simulink model "M10B39_es_V3"  (R2025a)
settings: Solver=ode23tb  StartTime=0.0  StopTime=100  FixedStep=0.001  MaxStep=0.01  RelTol=1e-3  EnableMultiTasking=on
InitFcn:
  | initAll_V3
values from neighbouring files (symbols this model uses):
  acom = 100    [initAll_V1.m]    (also in initAll_V2.m; initAll_V3.m; parameterinit.mat)
  AVm0 = [4.26082678503 4.656135219]    [parameterinit.mat]
  bcom = 50    [initAll_V1.m]    (also in initAll_V2.m; initAll_V3.m; parameterinit.mat)
  commun = 0*commun    [initAll_V1.m]    (also in initAll_V2.m; initAll_V3.m; parameterinit.mat = [0  0  0; 0  0  0; 0  0  0; 0  0  0])
  DataDelay = 0.0*DataDelay    [initAll_V1.m]    (also in initAll_V2.m; initAll_V3.m; parameterinit.mat = [0  0  0; 0  0  0; 0  0  0; 0  0  0])
  ESinit =     [parameterinit.mat]
  fB = 50    [initAll.m]    (also in initAll_V1.m; initAll_V2.m; initAll_V3.m; parameterinit.mat)
  Geninit = Generator_init(opdata,SynMach_in_gidx)    [initAll.m]    (also in initAll_V1.m; initAll_V2.m; initAll_V3.m = Generator_init(opdata_all,SynMach_in_gidx1); parameterinit.mat = )
  lam = 100    [initAll_V1.m]    (also in initAll_V2.m; initAll_V3.m; parameterinit.mat)
  SgridB = 100    [initAll.m]    (also in initAll_V1.m; initAll_V2.m; initAll_V3.m; parameterinit.mat)
  wB = 2*pi*fB    (= 314.159265359)    [initAll.m]    (also in initAll_V1.m; initAll_V2.m; initAll_V3.m; parameterinit.mat)
  Windinit =     [parameterinit.mat]
  YY_load = [3.65450097002 -2.05705688056 0 0 0 0 0 0 0 0 0 0 ... (1521 elements, 39x39)]    [parameterinit.mat]    (also in powerflowcaculate.m = full(YY))
undefined symbols (not defined in the file or in its folder): c1, c2, c3, c4, c5, c6, cp_nom, lambda_nom, P_wind_base, Pelec_base, Pnom
libraries: spsBistableLib x12, simulink_extras x3, slpidlib x2, simulink x1
(part 4 of 7)

== system M10B39_es_V3/Genrators/Generator1/Governor ==
  w : Inport
  Trip : Inport  Port=2
  CT : Constant  Value=0
  Constant : Constant  Value=0
  Gain : Gain  Gain=a_G  SaturateOnIntegerOverflow=on  OutDataTypeStr=Inherit: Same as input  ParamDataTypeStr=Inherit: Same as input
  Saturation : Saturate  UpperLimit=dPmax  LowerLimit=dPmin
  Sum1 : Sum  Inputs=|++  SaturateOnIntegerOverflow=on
  Sum3 : Sum  Inputs=|+-  SaturateOnIntegerOverflow=on
  Switch : Switch  Threshold=0.5  InputSameDT=off
  Switch1 : Switch  Criteria=u2 ~= 0  Threshold=0.5  InputSameDT=off
  Transfer Fcn1 : TransferFcn  Numerator=[b_G]  Denominator=[Tg_G 1]
  w0 : Gain  Gain=wB  SaturateOnIntegerOverflow=on  OutDataTypeStr=Inherit: Same as input  ParamDataTypeStr=Inherit: Same as input
  w1 : Constant  Value=S_Gov
  wref : Constant
  dPm : Outport
  wires:
  Gain/1 -> Sum1/1
  w1/1 -> Switch/2
  CT/1 -> Switch/3
  Sum3/1 -> w0/1
  Sum1/1 -> Saturation/1
  Saturation/1 -> Switch/1
  wref/1 -> Sum3/1
  w0/1 -> Gain/1, Transfer Fcn1/1
  Transfer Fcn1/1 -> Sum1/2
  w/1 -> Sum3/2
  Constant/1 -> Switch1/1
  Switch/1 -> Switch1/3
  Trip/1 -> Switch1/2
  Switch1/1 -> dPm/1

== system M10B39_es_V3/Genrators/Generator1/Machine Equations  ==
  note: Iqg
  note: Idg
  note: 接口
  delta : Inport
  Vgxy : Inport  Port=2
  Ef : Inport  Port=3
  Trip : Inport  Port=4
  Demux : Demux  Outputs=2
  Demux1 : Demux  Outputs=2
  Fcn1 : Fcn  Expr=u(1)*u(3)+u(2)*u(4)
  Fcn2 : Fcn  Expr=(u(3)-u(2))/Xd1
  Fcn3 : Fcn  Expr=(u(1)-u(4))/Xq1
  Fcn4 : Fcn  Expr=u(2)*u(3)-u(1)*u(4)
  Fcn6 : Fcn  Expr=sqrt(u(1)^2+u(2)^2)
  Interface : Subsystem
  Mux1 : Mux  Inputs=2
  Mux2 : Mux  Inputs=2
  Mux3 : Mux  Inputs=2
  Qe : Scope
      settings: TimeSpan=10  ActiveDisplayYMinimum=0.15  ActiveDisplayYMaximum=0.65
  Scope{,1..3} (4 alike) : Scope
      Scope settings: ActiveDisplayYMinimum=6.90941  ActiveDisplayYMaximum=6.93032
      Scope1 settings: ActiveDisplayYMinimum=0.73198  ActiveDisplayYMaximum=0.74189  DataLoggingVariableName=ScopeData2
      Scope2 settings: ActiveDisplayYMinimum=0.70724  ActiveDisplayYMaximum=0.71179  DataLoggingVariableName=ScopeData3
      Scope3 settings: ActiveDisplayYMinimum=3.59596  ActiveDisplayYMaximum=3.95434  DataLoggingVariableName=ScopeData4
  Transient Equations : Subsystem
  Pe : Outport
  Igxy1 : Outport  Port=2
  GBxy : Outport  Port=3
  Vg : Outport  Port=4
  wires:
  Trip/1 -> Transient Equations/3(Trip)
  Demux1/2 -> Scope3/1
  Demux/2 -> Scope2/1
  Demux1/1 -> Scope/1
  Demux/1 -> Scope1/1
  Transient Equations/1(Eqd') -> Interface/3(Eqd''), Mux1/2
  Interface/3(GBxy) -> GBxy/1
  Interface/2(Igxy1) -> Igxy1/1
  Vgxy/1 -> Interface/2(Vgxy)
  delta/1 -> Interface/1(delta)
  Fcn4/1 -> Qe/1
  Fcn6/1 -> Vg/1
  Fcn1/1 -> Pe/1
  Ef/1 -> Transient Equations/2(Ef)
  Mux2/1 -> Fcn4/1, Fcn1/1
  Mux1/1 -> Fcn3/1, Fcn2/1
  Interface/1(Vdqg) -> Mux1/1, Fcn6/1, Mux2/1, Demux/1
  Mux3/1 -> Mux2/2, Demux1/1, Transient Equations/1(Idqg)
  Fcn2/1 -> Mux3/1
  Fcn3/1 -> Mux3/2

== system M10B39_es_V3/Genrators/Generator1/Mechanical DE ==
  Pe : Inport
  dPm : Inport  Port=2
  Trip : Inport  Port=3
  Constant1 : Constant  Value=0
  Constant2 : Constant  Value=0
  Gain : Gain  Gain=wB  SaturateOnIntegerOverflow=on  OutDataTypeStr=Inherit: Same as input  ParamDataTypeStr=Inherit: Same as input
  Gain1 : Gain  Gain=1/H  SaturateOnIntegerOverflow=on  OutDataTypeStr=Inherit: Same as input  ParamDataTypeStr=Inherit: Same as input
  Gain2 : Gain  Gain=D  SaturateOnIntegerOverflow=on  OutDataTypeStr=Inherit: Same as input  ParamDataTypeStr=Inherit: Same as input
  Gain5 : Gain  Gain=180/pi  SaturateOnIntegerOverflow=on  OutDataTypeStr=Inherit: Same as input  ParamDataTypeStr=Inherit: Same as input
  Int1 : Integrator  InitialCondition=delta0
  Int2 : Integrator  InitialCondition=w0
  Pm : Constant  Value=Pm0
  Scope2 : Scope
      settings: TimeSpan=10  ActiveDisplayYMinimum=-0.4  ActiveDisplayYMaximum=1.4  DataLoggingVariableName=ScopeData5
  Scope4 : Scope
      settings: TimeSpan=10  ActiveDisplayYMinimum=0.99397  ActiveDisplayYMaximum=1.02044  DataLoggingVariableName=ScopeData6
  Scope8 : Scope
      settings: TimeSpan=10  ActiveDisplayYMinimum=-0.4  ActiveDisplayYMaximum=1.4  DataLoggingVariableName=ScopeData11
  Sum2 : Sum  Inputs=-+-+  SaturateOnIntegerOverflow=on
  Sum3 : Sum  Inputs=|+-  SaturateOnIntegerOverflow=on
  Switch{1..4} (4 alike) : Switch  Criteria=u2 ~= 0  Threshold=0.5  InputSameDT=off
  w0 : Constant
  delta : Outport
  w : Outport  Port=2
  wires:
  [Trip] -> Switch3/2, Switch2/2
  Constant1/1 -> Switch3/1, Switch2/1
  Switch3/1 -> Scope4/1, Sum3/1, w/1
  Int2/1 -> Switch3/3
  Switch2/1 -> Int2/1
  Gain1/1 -> Switch2/3
  Trip/1 -> [Trip]
  [Trip] -> Switch1/2, Switch4/2
  Constant2/1 -> Switch4/1, Switch1/1
  Switch4/1 -> delta/1, Scope2/1, Gain5/1
  Int1/1 -> Switch4/3
  Switch1/1 -> Int1/1
  Gain/1 -> Switch1/3
  Gain5/1 -> Scope8/1
  w0/1 -> Sum3/2
  Sum3/1 -> Gain2/1, Gain/1
  Pm/1 -> Sum2/2
  Gain2/1 -> Sum2/1
  Sum2/1 -> Gain1/1
  Pe/1 -> Sum2/3
  dPm/1 -> Sum2/4

== system M10B39_es_V3/Genrators/Generator1/Output ==
  Igxy1in : Inport
  GBxyin : Inport  Port=2
  deltain : Inport  Port=3
  Pein : Inport  Port=4
  fin : Inport  Port=5
  Vg : Inport  Port=6
  Bus Creator : BusCreator  Inputs=6
  m : Outport
  Igxy1 : Outport  Port=2
  GBxy : Outport  Port=3
  wires:
  Vg/1 -> Bus Creator/6  "Vg"
  fin/1 -> Bus Creator/5  "f"
  Pein/1 -> Bus Creator/4  "Pe"
  deltain/1 -> Bus Creator/3  "delta"
  GBxyin/1 -> Bus Creator/2, GBxy/1  "GBxy"
  Igxy1in/1 -> Bus Creator/1, Igxy1/1  "Igxy1"
  Bus Creator/1 -> m/1

== system M10B39_es_V3/Genrators/Generator1/PSS1 ==
  w : Inport
  Trip : Inport  Port=2
  CT : Constant  Value=0
  Constant : Constant  Value=0
  Gain : Gain  Gain=Kpss  SaturateOnIntegerOverflow=on  OutDataTypeStr=Inherit: Same as input  ParamDataTypeStr=Inherit: Same as input
  Saturation : Saturate  UpperLimit=Upmax  LowerLimit=Upmin
  Sum3 : Sum  Inputs=|+-  SaturateOnIntegerOverflow=on
  Switch : Switch  Threshold=0.5  InputSameDT=off
  Switch1 : Switch  Threshold=0.5  InputSameDT=off
  Transfer Fcn : TransferFcn  Numerator=[Tw_P 0]  Denominator=[Tw_P 1]
  Transfer Fcn1 : TransferFcn  Numerator=[T1_P 1]  Denominator=[T2_P 1]
  Transfer Fcn2 : TransferFcn  Numerator=[T3_P 1]  Denominator=[T4_P 1]
  w0 : Constant
  w1 : Constant  Value=S_PSS
  Upss : Outport
  wires:
  Constant/1 -> Switch1/1
  Trip/1 -> Switch1/2
  Switch1/1 -> Upss/1
  Switch/1 -> Switch1/3
  Transfer Fcn/1 -> Transfer Fcn1/1
  Gain/1 -> Transfer Fcn/1
  w1/1 -> Switch/2
  CT/1 -> Switch/3
  Saturation/1 -> Switch/1
  Sum3/1 -> Gain/1
  Transfer Fcn2/1 -> Saturation/1
  Transfer Fcn1/1 -> Transfer Fcn2/1
  w/1 -> Sum3/1
  w0/1 -> Sum3/2

== system M10B39_es_V3/Genrators/Generator10/Excitation System ST1A1 ==
  note: Ef
  Upss : Inport
  Trip : Inport  Port=2
  Vg : Inport  Port=3
  Constant1 : Constant  Value=0
  Ef1 : Integrator  InitialCondition=Ef10
  K : Gain  Gain=1/Tb  SaturateOnIntegerOverflow=on  OutDataTypeStr=Inherit: Same as input  ParamDataTypeStr=Inherit: Same as input
  KA : Gain  Gain=Ka  SaturateOnIntegerOverflow=on  OutDataTypeStr=Inherit: Same as input  ParamDataTypeStr=Inherit: Same as input
  KA1 : Gain  Gain=Tc/Tb  SaturateOnIntegerOverflow=on  OutDataTypeStr=Inherit: Same as input  ParamDataTypeStr=Inherit: Same as input
  KA2 : Gain  Gain=(1/Tb)*(1-Tc/Tb)  SaturateOnIntegerOverflow=on  OutDataTypeStr=Inherit: Same as input  ParamDataTypeStr=Inherit: Same as input
  Saturation : Saturate  UpperLimit=Efmax  LowerLimit=Efmin
  Sum : Sum  Inputs=|++  SaturateOnIntegerOverflow=on
  Sum1 : Sum  Inputs=|+-  SaturateOnIntegerOverflow=on
  Sum4 : Sum  Inputs=|+-+  SaturateOnIntegerOverflow=on
  Switch2 : Switch  Criteria=u2 ~= 0  Threshold=0.5  InputSameDT=off
  Switch3 : Switch  Criteria=u2 ~= 0  Threshold=0.5  InputSameDT=off
  Vref : Constant  Value=Vref
  Ef : Outport
  wires:
  Trip/1 -> Switch3/2, Switch2/2
  Constant1/1 -> Switch3/1, Switch2/1
  Switch3/1 -> KA2/1, K/1
  Ef1/1 -> Switch3/3
  Switch2/1 -> Ef1/1
  Sum1/1 -> Switch2/3
  KA/1 -> KA1/1, Sum1/1
  Upss/1 -> Sum4/3
  Saturation/1 -> Ef/1
  Vg/1 -> Sum4/2
  Sum4/1 -> KA/1
  Vref/1 -> Sum4/1
  Sum/1 -> Saturation/1
  K/1 -> Sum1/2
  KA1/1 -> Sum/2
  KA2/1 -> Sum/1

== system M10B39_es_V3/Genrators/Generator10/Governor ==
  w : Inport
  Trip : Inport  Port=2
  CT : Constant  Value=0
  Constant : Constant  Value=0
  Gain : Gain  Gain=a_G  SaturateOnIntegerOverflow=on  OutDataTypeStr=Inherit: Same as input  ParamDataTypeStr=Inherit: Same as input
  Saturation : Saturate  UpperLimit=dPmax  LowerLimit=dPmin
  Sum1 : Sum  Inputs=|++  SaturateOnIntegerOverflow=on
  Sum3 : Sum  Inputs=|+-  SaturateOnIntegerOverflow=on
  Switch : Switch  Threshold=0.5  InputSameDT=off
  Switch1 : Switch  Criteria=u2 ~= 0  Threshold=0.5  InputSameDT=off
  Transfer Fcn1 : TransferFcn  Numerator=[b_G]  Denominator=[Tg_G 1]
  w0 : Gain  Gain=wB  SaturateOnIntegerOverflow=on  OutDataTypeStr=Inherit: Same as input  ParamDataTypeStr=Inherit: Same as input
  w1 : Constant  Value=S_Gov
  wref : Constant
  dPm : Outport
  wires:
  Gain/1 -> Sum1/1
  w1/1 -> Switch/2
  CT/1 -> Switch/3
  Sum3/1 -> w0/1
  Sum1/1 -> Saturation/1
  Saturation/1 -> Switch/1
  wref/1 -> Sum3/1
  w0/1 -> Gain/1, Transfer Fcn1/1
  Transfer Fcn1/1 -> Sum1/2
  w/1 -> Sum3/2
  Constant/1 -> Switch1/1
  Switch/1 -> Switch1/3
  Trip/1 -> Switch1/2
  Switch1/1 -> dPm/1

== system M10B39_es_V3/Genrators/Generator10/Machine Equations  ==
  note: Iqg
  note: Idg
  note: 接口
  delta : Inport
  Vgxy : Inport  Port=2
  Ef : Inport  Port=3
  Trip : Inport  Port=4
  Demux : Demux  Outputs=2
  Demux1 : Demux  Outputs=2
  Fcn1 : Fcn  Expr=u(1)*u(3)+u(2)*u(4)
  Fcn2 : Fcn  Expr=(u(3)-u(2))/Xd1
  Fcn3 : Fcn  Expr=(u(1)-u(4))/Xq1
  Fcn4 : Fcn  Expr=u(2)*u(3)-u(1)*u(4)
  Fcn6 : Fcn  Expr=sqrt(u(1)^2+u(2)^2)
  Interface : Subsystem
  Mux1 : Mux  Inputs=2
  Mux2 : Mux  Inputs=2
  Mux3 : Mux  Inputs=2
  Qe : Scope
      settings: TimeSpan=10  ActiveDisplayYMinimum=0.15  ActiveDisplayYMaximum=0.65
  Scope{,1..3} (4 alike) : Scope
      Scope settings: ActiveDisplayYMinimum=6.90941  ActiveDisplayYMaximum=6.93032
      Scope1 settings: ActiveDisplayYMinimum=0.73198  ActiveDisplayYMaximum=0.74189  DataLoggingVariableName=ScopeData2
      Scope2 settings: ActiveDisplayYMinimum=0.70724  ActiveDisplayYMaximum=0.71179  DataLoggingVariableName=ScopeData3
      Scope3 settings: ActiveDisplayYMinimum=3.59596  ActiveDisplayYMaximum=3.95434  DataLoggingVariableName=ScopeData4
  Transient Equations : Subsystem
  Pe : Outport
  Igxy1 : Outport  Port=2
  GBxy : Outport  Port=3
  Vg : Outport  Port=4
  wires:
  Trip/1 -> Transient Equations/3(Trip)
  Demux1/2 -> Scope3/1
  Demux/2 -> Scope2/1
  Demux1/1 -> Scope/1
  Demux/1 -> Scope1/1
  Transient Equations/1(Eqd') -> Interface/3(Eqd''), Mux1/2
  Interface/3(GBxy) -> GBxy/1
  Interface/2(Igxy1) -> Igxy1/1
  Vgxy/1 -> Interface/2(Vgxy)
  delta/1 -> Interface/1(delta)
  Fcn4/1 -> Qe/1
  Fcn6/1 -> Vg/1
  Fcn1/1 -> Pe/1
  Ef/1 -> Transient Equations/2(Ef)
  Mux2/1 -> Fcn4/1, Fcn1/1
  Mux1/1 -> Fcn3/1, Fcn2/1
  Interface/1(Vdqg) -> Mux1/1, Fcn6/1, Mux2/1, Demux/1
  Mux3/1 -> Mux2/2, Demux1/1, Transient Equations/1(Idqg)
  Fcn2/1 -> Mux3/1
  Fcn3/1 -> Mux3/2

== system M10B39_es_V3/Genrators/Generator10/Mechanical DE ==
  Pe : Inport
  dPm : Inport  Port=2
  Trip : Inport  Port=3
  Constant1 : Constant  Value=0
  Constant2 : Constant  Value=0
  Gain : Gain  Gain=wB  SaturateOnIntegerOverflow=on  OutDataTypeStr=Inherit: Same as input  ParamDataTypeStr=Inherit: Same as input
  Gain1 : Gain  Gain=1/H  SaturateOnIntegerOverflow=on  OutDataTypeStr=Inherit: Same as input  ParamDataTypeStr=Inherit: Same as input
  Gain2 : Gain  Gain=D  SaturateOnIntegerOverflow=on  OutDataTypeStr=Inherit: Same as input  ParamDataTypeStr=Inherit: Same as input
  Gain5 : Gain  Gain=180/pi  SaturateOnIntegerOverflow=on  OutDataTypeStr=Inherit: Same as input  ParamDataTypeStr=Inherit: Same as input
  Int1 : Integrator  InitialCondition=delta0
  Int2 : Integrator  InitialCondition=w0
  Pm : Constant  Value=Pm0
  Scope2 : Scope
      settings: TimeSpan=10  ActiveDisplayYMinimum=-0.4  ActiveDisplayYMaximum=1.4  DataLoggingVariableName=ScopeData5
  Scope4 : Scope
      settings: TimeSpan=10  ActiveDisplayYMinimum=0.99397  ActiveDisplayYMaximum=1.02044  DataLoggingVariableName=ScopeData6
  Scope8 : Scope
      settings: TimeSpan=10  ActiveDisplayYMinimum=-0.4  ActiveDisplayYMaximum=1.4  DataLoggingVariableName=ScopeData11
  Sum2 : Sum  Inputs=-+-+  SaturateOnIntegerOverflow=on
  Sum3 : Sum  Inputs=|+-  SaturateOnIntegerOverflow=on
  Switch{1..4} (4 alike) : Switch  Criteria=u2 ~= 0  Threshold=0.5  InputSameDT=off
  w0 : Constant
  delta : Outport
  w : Outport  Port=2
  wires:
  [Trip] -> Switch3/2, Switch2/2
  Constant1/1 -> Switch3/1, Switch2/1
  Switch3/1 -> Scope4/1, Sum3/1, w/1
  Int2/1 -> Switch3/3
  Switch2/1 -> Int2/1
  Gain1/1 -> Switch2/3
  Trip/1 -> [Trip]
  [Trip] -> Switch1/2, Switch4/2
  Constant2/1 -> Switch4/1, Switch1/1
  Switch4/1 -> delta/1, Scope2/1, Gain5/1
  Int1/1 -> Switch4/3
  Switch1/1 -> Int1/1
  Gain/1 -> Switch1/3
  Gain5/1 -> Scope8/1
  w0/1 -> Sum3/2
  Sum3/1 -> Gain2/1, Gain/1
  Pm/1 -> Sum2/2
  Gain2/1 -> Sum2/1
  Sum2/1 -> Gain1/1
  Pe/1 -> Sum2/3
  dPm/1 -> Sum2/4

== system M10B39_es_V3/Genrators/Generator10/Output ==
  Igxy1in : Inport
  GBxyin : Inport  Port=2
  deltain : Inport  Port=3
  Pein : Inport  Port=4
  fin : Inport  Port=5
  Vg : Inport  Port=6
  Bus Creator : BusCreator  Inputs=6
  m : Outport
  Igxy1 : Outport  Port=2
  GBxy : Outport  Port=3
  wires:
  Vg/1 -> Bus Creator/6  "Vg"
  fin/1 -> Bus Creator/5  "f"
  Pein/1 -> Bus Creator/4  "Pe"
  deltain/1 -> Bus Creator/3  "delta"
  GBxyin/1 -> Bus Creator/2, GBxy/1  "GBxy"
  Igxy1in/1 -> Bus Creator/1, Igxy1/1  "Igxy1"
  Bus Creator/1 -> m/1

== system M10B39_es_V3/Genrators/Generator10/PSS1 ==
  w : Inport
  Trip : Inport  Port=2
  CT : Constant  Value=0
  Constant : Constant  Value=0
  Gain : Gain  Gain=Kpss  SaturateOnIntegerOverflow=on  OutDataTypeStr=Inherit: Same as input  ParamDataTypeStr=Inherit: Same as input
  Saturation : Saturate  UpperLimit=Upmax  LowerLimit=Upmin
  Sum3 : Sum  Inputs=|+-  SaturateOnIntegerOverflow=on
  Switch : Switch  Threshold=0.5  InputSameDT=off
  Switch1 : Switch  Threshold=0.5  InputSameDT=off
  Transfer Fcn : TransferFcn  Numerator=[Tw_P 0]  Denominator=[Tw_P 1]
  Transfer Fcn1 : TransferFcn  Numerator=[T1_P 1]  Denominator=[T2_P 1]
  Transfer Fcn2 : TransferFcn  Numerator=[T3_P 1]  Denominator=[T4_P 1]
  w0 : Constant
  w1 : Constant  Value=S_PSS
  Upss : Outport
  wires:
  Constant/1 -> Switch1/1
  Trip/1 -> Switch1/2
  Switch1/1 -> Upss/1
  Switch/1 -> Switch1/3
  Transfer Fcn/1 -> Transfer Fcn1/1
  Gain/1 -> Transfer Fcn/1
  w1/1 -> Switch/2
  CT/1 -> Switch/3
  Saturation/1 -> Switch/1
  Sum3/1 -> Gain/1
  Transfer Fcn2/1 -> Saturation/1
  Transfer Fcn1/1 -> Transfer Fcn2/1
  w/1 -> Sum3/1
  w0/1 -> Sum3/2

== system M10B39_es_V3/Genrators/Generator3/Excitation System ST1A1 ==
  note: Ef
  Upss : Inport
  Trip : Inport  Port=2
  Vg : Inport  Port=3
  Constant1 : Constant  Value=0
  Ef1 : Integrator  InitialCondition=Ef10
  K : Gain  Gain=1/Tb  SaturateOnIntegerOverflow=on  OutDataTypeStr=Inherit: Same as input  ParamDataTypeStr=Inherit: Same as input
  KA : Gain  Gain=Ka  SaturateOnIntegerOverflow=on  OutDataTypeStr=Inherit: Same as input  ParamDataTypeStr=Inherit: Same as input
  KA1 : Gain  Gain=Tc/Tb  SaturateOnIntegerOverflow=on  OutDataTypeStr=Inherit: Same as input  ParamDataTypeStr=Inherit: Same as input
  KA2 : Gain  Gain=(1/Tb)*(1-Tc/Tb)  SaturateOnIntegerOverflow=on  OutDataTypeStr=Inherit: Same as input  ParamDataTypeStr=Inherit: Same as input
  Saturation : Saturate  UpperLimit=Efmax  LowerLimit=Efmin
  Sum : Sum  Inputs=|++  SaturateOnIntegerOverflow=on
  Sum1 : Sum  Inputs=|+-  SaturateOnIntegerOverflow=on
  Sum4 : Sum  Inputs=|+-+  SaturateOnIntegerOverflow=on
  Switch2 : Switch  Criteria=u2 ~= 0  Threshold=0.5  InputSameDT=off
  Switch3 : Switch  Criteria=u2 ~= 0  Threshold=0.5  InputSameDT=off
  Vref : Constant  Value=Vref
  Ef : Outport
  wires:
  Trip/1 -> Switch3/2, Switch2/2
  Constant1/1 -> Switch3/1, Switch2/1
  Switch3/1 -> KA2/1, K/1
  Ef1/1 -> Switch3/3
  Switch2/1 -> Ef1/1
  Sum1/1 -> Switch2/3
  KA/1 -> KA1/1, Sum1/1
  Upss/1 -> Sum4/3
  Saturation/1 -> Ef/1
  Vg/1 -> Sum4/2
  Sum4/1 -> KA/1
  Vref/1 -> Sum4/1
  Sum/1 -> Saturation/1
  K/1 -> Sum1/2
  KA1/1 -> Sum/2
  KA2/1 -> Sum/1

== system M10B39_es_V3/Genrators/Generator3/Governor ==
  w : Inport
  Trip : Inport  Port=2
  CT : Constant  Value=0
  Constant : Constant  Value=0
  Gain : Gain  Gain=a_G  SaturateOnIntegerOverflow=on  OutDataTypeStr=Inherit: Same as input  ParamDataTypeStr=Inherit: Same as input
  Saturation : Saturate  UpperLimit=dPmax  LowerLimit=dPmin
  Sum1 : Sum  Inputs=|++  SaturateOnIntegerOverflow=on
  Sum3 : Sum  Inputs=|+-  SaturateOnIntegerOverflow=on
  Switch : Switch  Threshold=0.5  InputSameDT=off
  Switch1 : Switch  Criteria=u2 ~= 0  Threshold=0.5  InputSameDT=off
  Transfer Fcn1 : TransferFcn  Numerator=[b_G]  Denominator=[Tg_G 1]
  w0 : Gain  Gain=wB  SaturateOnIntegerOverflow=on  OutDataTypeStr=Inherit: Same as input  ParamDataTypeStr=Inherit: Same as input
  w1 : Constant  Value=S_Gov
  wref : Constant
  dPm : Outport
  wires:
  Gain/1 -> Sum1/1
  w1/1 -> Switch/2
  CT/1 -> Switch/3
  Sum3/1 -> w0/1
  Sum1/1 -> Saturation/1
  Saturation/1 -> Switch/1
  wref/1 -> Sum3/1
  w0/1 -> Gain/1, Transfer Fcn1/1
  Transfer Fcn1/1 -> Sum1/2
  w/1 -> Sum3/2
  Constant/1 -> Switch1/1
  Switch/1 -> Switch1/3
  Trip/1 -> Switch1/2
  Switch1/1 -> dPm/1

== system M10B39_es_V3/Genrators/Generator3/Machine Equations  ==
  note: Iqg
  note: Idg
  note: 接口
  delta : Inport
  Vgxy : Inport  Port=2
  Ef : Inport  Port=3
  Trip : Inport  Port=4
  Demux : Demux  Outputs=2
  Demux1 : Demux  Outputs=2
  Fcn1 : Fcn  Expr=u(1)*u(3)+u(2)*u(4)
  Fcn2 : Fcn  Expr=(u(3)-u(2))/Xd1
  Fcn3 : Fcn  Expr=(u(1)-u(4))/Xq1
  Fcn4 : Fcn  Expr=u(2)*u(3)-u(1)*u(4)
  Fcn6 : Fcn  Expr=sqrt(u(1)^2+u(2)^2)
  Interface : Subsystem
  Mux1 : Mux  Inputs=2
  Mux2 : Mux  Inputs=2
  Mux3 : Mux  Inputs=2
  Qe : Scope
      settings: TimeSpan=10  ActiveDisplayYMinimum=0.15  ActiveDisplayYMaximum=0.65
  Scope{,1..3} (4 alike) : Scope
      Scope settings: ActiveDisplayYMinimum=6.90941  ActiveDisplayYMaximum=6.93032
      Scope1 settings: ActiveDisplayYMinimum=0.73198  ActiveDisplayYMaximum=0.74189  DataLoggingVariableName=ScopeData2
      Scope2 settings: ActiveDisplayYMinimum=0.70724  ActiveDisplayYMaximum=0.71179  DataLoggingVariableName=ScopeData3
      Scope3 settings: ActiveDisplayYMinimum=3.59596  ActiveDisplayYMaximum=3.95434  DataLoggingVariableName=ScopeData4
  Transient Equations : Subsystem
  Pe : Outport
  Igxy1 : Outport  Port=2
  GBxy : Outport  Port=3
  Vg : Outport  Port=4
  wires:
  Trip/1 -> Transient Equations/3(Trip)
  Demux1/2 -> Scope3/1
  Demux/2 -> Scope2/1
  Demux1/1 -> Scope/1
  Demux/1 -> Scope1/1
  Transient Equations/1(Eqd') -> Interface/3(Eqd''), Mux1/2
  Interface/3(GBxy) -> GBxy/1
  Interface/2(Igxy1) -> Igxy1/1
  Vgxy/1 -> Interface/2(Vgxy)
  delta/1 -> Interface/1(delta)
  Fcn4/1 -> Qe/1
  Fcn6/1 -> Vg/1
  Fcn1/1 -> Pe/1
  Ef/1 -> Transient Equations/2(Ef)
  Mux2/1 -> Fcn4/1, Fcn1/1
  Mux1/1 -> Fcn3/1, Fcn2/1
  Interface/1(Vdqg) -> Mux1/1, Fcn6/1, Mux2/1, Demux/1
  Mux3/1 -> Mux2/2, Demux1/1, Transient Equations/1(Idqg)
  Fcn2/1 -> Mux3/1
  Fcn3/1 -> Mux3/2

== system M10B39_es_V3/Genrators/Generator3/Mechanical DE ==
  Pe : Inport
  dPm : Inport  Port=2
  Trip : Inport  Port=3
  Constant1 : Constant  Value=0
  Constant2 : Constant  Value=0
  Gain : Gain  Gain=wB  SaturateOnIntegerOverflow=on  OutDataTypeStr=Inherit: Same as input  ParamDataTypeStr=Inherit: Same as input
  Gain1 : Gain  Gain=1/H  SaturateOnIntegerOverflow=on  OutDataTypeStr=Inherit: Same as input  ParamDataTypeStr=Inherit: Same as input
  Gain2 : Gain  Gain=D  SaturateOnIntegerOverflow=on  OutDataTypeStr=Inherit: Same as input  ParamDataTypeStr=Inherit: Same as input
  Gain5 : Gain  Gain=180/pi  SaturateOnIntegerOverflow=on  OutDataTypeStr=Inherit: Same as input  ParamDataTypeStr=Inherit: Same as input
  Int1 : Integrator  InitialCondition=delta0
  Int2 : Integrator  InitialCondition=w0
  Pm : Constant  Value=Pm0
  Scope2 : Scope
      settings: TimeSpan=10  ActiveDisplayYMinimum=-0.4  ActiveDisplayYMaximum=1.4  DataLoggingVariableName=ScopeData5
  Scope4 : Scope
      settings: TimeSpan=10  ActiveDisplayYMinimum=0.99397  ActiveDisplayYMaximum=1.02044  DataLoggingVariableName=ScopeData6
  Scope8 : Scope
      settings: TimeSpan=10  ActiveDisplayYMinimum=-0.4  ActiveDisplayYMaximum=1.4  DataLoggingVariableName=ScopeData11
  Sum2 : Sum  Inputs=-+-+  SaturateOnIntegerOverflow=on
  Sum3 : Sum  Inputs=|+-  SaturateOnIntegerOverflow=on
  Switch{1..4} (4 alike) : Switch  Criteria=u2 ~= 0  Threshold=0.5  InputSameDT=off
  w0 : Constant
  delta : Outport
  w : Outport  Port=2
  wires:
  [Trip] -> Switch3/2, Switch2/2
  Constant1/1 -> Switch3/1, Switch2/1
  Switch3/1 -> Scope4/1, Sum3/1, w/1
  Int2/1 -> Switch3/3
  Switch2/1 -> Int2/1
  Gain1/1 -> Switch2/3
  Trip/1 -> [Trip]
  [Trip] -> Switch1/2, Switch4/2
  Constant2/1 -> Switch4/1, Switch1/1
  Switch4/1 -> delta/1, Scope2/1, Gain5/1
  Int1/1 -> Switch4/3
  Switch1/1 -> Int1/1
  Gain/1 -> Switch1/3
  Gain5/1 -> Scope8/1
  w0/1 -> Sum3/2
  Sum3/1 -> Gain2/1, Gain/1
  Pm/1 -> Sum2/2
  Gain2/1 -> Sum2/1
  Sum2/1 -> Gain1/1
  Pe/1 -> Sum2/3
  dPm/1 -> Sum2/4

== system M10B39_es_V3/Genrators/Generator3/Output ==
  Igxy1in : Inport
  GBxyin : Inport  Port=2
  deltain : Inport  Port=3
  Pein : Inport  Port=4
  fin : Inport  Port=5
  Vg : Inport  Port=6
  Bus Creator : BusCreator  Inputs=6
  m : Outport
  Igxy1 : Outport  Port=2
  GBxy : Outport  Port=3
  wires:
  Vg/1 -> Bus Creator/6  "Vg"
  fin/1 -> Bus Creator/5  "f"
  Pein/1 -> Bus Creator/4  "Pe"
  deltain/1 -> Bus Creator/3  "delta"
  GBxyin/1 -> Bus Creator/2, GBxy/1  "GBxy"
  Igxy1in/1 -> Bus Creator/1, Igxy1/1  "Igxy1"
  Bus Creator/1 -> m/1

== system M10B39_es_V3/Genrators/Generator3/PSS1 ==
  w : Inport
  Trip : Inport  Port=2
  CT : Constant  Value=0
  Constant : Constant  Value=0
  Gain : Gain  Gain=Kpss  SaturateOnIntegerOverflow=on  OutDataTypeStr=Inherit: Same as input  ParamDataTypeStr=Inherit: Same as input
  Saturation : Saturate  UpperLimit=Upmax  LowerLimit=Upmin
  Sum3 : Sum  Inputs=|+-  SaturateOnIntegerOverflow=on
  Switch : Switch  Threshold=0.5  InputSameDT=off
  Switch1 : Switch  Threshold=0.5  InputSameDT=off
  Transfer Fcn : TransferFcn  Numerator=[Tw_P 0]  Denominator=[Tw_P 1]
  Transfer Fcn1 : TransferFcn  Numerator=[T1_P 1]  Denominator=[T2_P 1]
  Transfer Fcn2 : TransferFcn  Numerator=[T3_P 1]  Denominator=[T4_P 1]
  w0 : Constant
  w1 : Constant  Value=S_PSS
  Upss : Outport
  wires:
  Constant/1 -> Switch1/1
  Trip/1 -> Switch1/2
  Switch1/1 -> Upss/1
  Switch/1 -> Switch1/3
  Transfer Fcn/1 -> Transfer Fcn1/1
  Gain/1 -> Transfer Fcn/1
  w1/1 -> Switch/2
  CT/1 -> Switch/3
  Saturation/1 -> Switch/1
  Sum3/1 -> Gain/1
  Transfer Fcn2/1 -> Saturation/1
  Transfer Fcn1/1 -> Transfer Fcn2/1
  w/1 -> Sum3/1
  w0/1 -> Sum3/2

== system M10B39_es_V3/Genrators/Generator4/Excitation System ST1A1 ==
  note: Ef
  Upss : Inport
  Trip : Inport  Port=2
  Vg : Inport  Port=3
  Constant1 : Constant  Value=0
  Ef1 : Integrator  InitialCondition=Ef10
  K : Gain  Gain=1/Tb  SaturateOnIntegerOverflow=on  OutDataTypeStr=Inherit: Same as input  ParamDataTypeStr=Inherit: Same as input
  KA : Gain  Gain=Ka  SaturateOnIntegerOverflow=on  OutDataTypeStr=Inherit: Same as input  ParamDataTypeStr=Inherit: Same as input
  KA1 : Gain  Gain=Tc/Tb  SaturateOnIntegerOverflow=on  OutDataTypeStr=Inherit: Same as input  ParamDataTypeStr=Inherit: Same as input
  KA2 : Gain  Gain=(1/Tb)*(1-Tc/Tb)  SaturateOnIntegerOverflow=on  OutDataTypeStr=Inherit: Same as input  ParamDataTypeStr=Inherit: Same as input
  Saturation : Saturate  UpperLimit=Efmax  LowerLimit=Efmin
  Sum : Sum  Inputs=|++  SaturateOnIntegerOverflow=on
  Sum1 : Sum  Inputs=|+-  SaturateOnIntegerOverflow=on
  Sum4 : Sum  Inputs=|+-+  SaturateOnIntegerOverflow=on
  Switch2 : Switch  Criteria=u2 ~= 0  Threshold=0.5  InputSameDT=off
  Switch3 : Switch  Criteria=u2 ~= 0  Threshold=0.5  InputSameDT=off
  Vref : Constant  Value=Vref
  Ef : Outport
  wires:
  Trip/1 -> Switch3/2, Switch2/2
  Constant1/1 -> Switch3/1, Switch2/1
  Switch3/1 -> KA2/1, K/1
  Ef1/1 -> Switch3/3
  Switch2/1 -> Ef1/1
  Sum1/1 -> Switch2/3
  KA/1 -> KA1/1, Sum1/1
  Upss/1 -> Sum4/3
  Saturation/1 -> Ef/1
  Vg/1 -> Sum4/2
  Sum4/1 -> KA/1
  Vref/1 -> Sum4/1
  Sum/1 -> Saturation/1
  K/1 -> Sum1/2
  KA1/1 -> Sum/2
  KA2/1 -> Sum/1

== system M10B39_es_V3/Genrators/Generator4/Governor ==
  w : Inport
  Trip : Inport  Port=2
  CT : Constant  Value=0
  Constant : Constant  Value=0
  Gain : Gain  Gain=a_G  SaturateOnIntegerOverflow=on  OutDataTypeStr=Inherit: Same as input  ParamDataTypeStr=Inherit: Same as input
  Saturation : Saturate  UpperLimit=dPmax  LowerLimit=dPmin
  Sum1 : Sum  Inputs=|++  SaturateOnIntegerOverflow=on
  Sum3 : Sum  Inputs=|+-  SaturateOnIntegerOverflow=on
  Switch : Switch  Threshold=0.5  InputSameDT=off
  Switch1 : Switch  Criteria=u2 ~= 0  Threshold=0.5  InputSameDT=off
  Transfer Fcn1 : TransferFcn  Numerator=[b_G]  Denominator=[Tg_G 1]
  w0 : Gain  Gain=wB  SaturateOnIntegerOverflow=on  OutDataTypeStr=Inherit: Same as input  ParamDataTypeStr=Inherit: Same as input
  w1 : Constant  Value=S_Gov
  wref : Constant
  dPm : Outport
  wires:
  Gain/1 -> Sum1/1
  w1/1 -> Switch/2
  CT/1 -> Switch/3
  Sum3/1 -> w0/1
  Sum1/1 -> Saturation/1
  Saturation/1 -> Switch/1
  wref/1 -> Sum3/1
  w0/1 -> Gain/1, Transfer Fcn1/1
  Transfer Fcn1/1 -> Sum1/2
  w/1 -> Sum3/2
  Constant/1 -> Switch1/1
  Switch/1 -> Switch1/3
  Trip/1 -> Switch1/2
  Switch1/1 -> dPm/1

== system M10B39_es_V3/Genrators/Generator4/Machine Equations  ==
  note: Iqg
  note: Idg
  note: 接口
  delta : Inport
  Vgxy : Inport  Port=2
  Ef : Inport  Port=3
  Trip : Inport  Port=4
  Demux : Demux  Outputs=2
  Demux1 : Demux  Outputs=2
  Fcn1 : Fcn  Expr=u(1)*u(3)+u(2)*u(4)
  Fcn2 : Fcn  Expr=(u(3)-u(2))/Xd1
  Fcn3 : Fcn  Expr=(u(1)-u(4))/Xq1
  Fcn4 : Fcn  Expr=u(2)*u(3)-u(1)*u(4)
  Fcn6 : Fcn  Expr=sqrt(u(1)^2+u(2)^2)
  Interface : Subsystem
  Mux1 : Mux  Inputs=2
  Mux2 : Mux  Inputs=2
  Mux3 : Mux  Inputs=2
  Qe : Scope
      settings: TimeSpan=10  ActiveDisplayYMinimum=0.15  ActiveDisplayYMaximum=0.65
  Scope{,1..3} (4 alike) : Scope
      Scope settings: ActiveDisplayYMinimum=6.90941  ActiveDisplayYMaximum=6.93032
      Scope1 settings: ActiveDisplayYMinimum=0.73198  ActiveDisplayYMaximum=0.74189  DataLoggingVariableName=ScopeData2
      Scope2 settings: ActiveDisplayYMinimum=0.70724  ActiveDisplayYMaximum=0.71179  DataLoggingVariableName=ScopeData3
      Scope3 settings: ActiveDisplayYMinimum=3.59596  ActiveDisplayYMaximum=3.95434  DataLoggingVariableName=ScopeData4
  Transient Equations : Subsystem
  Pe : Outport
  Igxy1 : Outport  Port=2
  GBxy : Outport  Port=3
  Vg : Outport  Port=4
  wires:
  Trip/1 -> Transient Equations/3(Trip)
  Demux1/2 -> Scope3/1
  Demux/2 -> Scope2/1
  Demux1/1 -> Scope/1
  Demux/1 -> Scope1/1
  Transient Equations/1(Eqd') -> Interface/3(Eqd''), Mux1/2
  Interface/3(GBxy) -> GBxy/1
  Interface/2(Igxy1) -> Igxy1/1
  Vgxy/1 -> Interface/2(Vgxy)
  delta/1 -> Interface/1(delta)
  Fcn4/1 -> Qe/1
  Fcn6/1 -> Vg/1
  Fcn1/1 -> Pe/1
  Ef/1 -> Transient Equations/2(Ef)
  Mux2/1 -> Fcn4/1, Fcn1/1
  Mux1/1 -> Fcn3/1, Fcn2/1
  Interface/1(Vdqg) -> Mux1/1, Fcn6/1, Mux2/1, Demux/1
  Mux3/1 -> Mux2/2, Demux1/1, Transient Equations/1(Idqg)
  Fcn2/1 -> Mux3/1
  Fcn3/1 -> Mux3/2

== system M10B39_es_V3/Genrators/Generator4/Mechanical DE ==
  Pe : Inport
  dPm : Inport  Port=2
  Trip : Inport  Port=3
  Constant1 : Constant  Value=0
  Constant2 : Constant  Value=0
  Gain : Gain  Gain=wB  SaturateOnIntegerOverflow=on  OutDataTypeStr=Inherit: Same as input  ParamDataTypeStr=Inherit: Same as input
  Gain1 : Gain  Gain=1/H  SaturateOnIntegerOverflow=on  OutDataTypeStr=Inherit: Same as input  ParamDataTypeStr=Inherit: Same as input
  Gain2 : Gain  Gain=D  SaturateOnIntegerOverflow=on  OutDataTypeStr=Inherit: Same as input  ParamDataTypeStr=Inherit: Same as input
  Gain5 : Gain  Gain=180/pi  SaturateOnIntegerOverflow=on  OutDataTypeStr=Inherit: Same as input  ParamDataTypeStr=Inherit: Same as input
  Int1 : Integrator  InitialCondition=delta0
  Int2 : Integrator  InitialCondition=w0
  Pm : Constant  Value=Pm0
  Scope2 : Scope
      settings: TimeSpan=10  ActiveDisplayYMinimum=-0.4  ActiveDisplayYMaximum=1.4  DataLoggingVariableName=ScopeData5
  Scope4 : Scope
      settings: TimeSpan=10  ActiveDisplayYMinimum=0.99397  ActiveDisplayYMaximum=1.02044  DataLoggingVariableName=ScopeData6
  Scope8 : Scope
      settings: TimeSpan=10  ActiveDisplayYMinimum=-0.4  ActiveDisplayYMaximum=1.4  DataLoggingVariableName=ScopeData11
  Sum2 : Sum  Inputs=-+-+  SaturateOnIntegerOverflow=on
  Sum3 : Sum  Inputs=|+-  SaturateOnIntegerOverflow=on
  Switch{1..4} (4 alike) : Switch  Criteria=u2 ~= 0  Threshold=0.5  InputSameDT=off
  w0 : Constant
  delta : Outport
  w : Outport  Port=2
  wires:
  [Trip] -> Switch3/2, Switch2/2
  Constant1/1 -> Switch3/1, Switch2/1
  Switch3/1 -> Scope4/1, Sum3/1, w/1
  Int2/1 -> Switch3/3
  Switch2/1 -> Int2/1
  Gain1/1 -> Switch2/3
  Trip/1 -> [Trip]
  [Trip] -> Switch1/2, Switch4/2
  Constant2/1 -> Switch4/1, Switch1/1
  Switch4/1 -> delta/1, Scope2/1, Gain5/1
  Int1/1 -> Switch4/3
  Switch1/1 -> Int1/1
  Gain/1 -> Switch1/3
  Gain5/1 -> Scope8/1
  w0/1 -> Sum3/2
  Sum3/1 -> Gain2/1, Gain/1
  Pm/1 -> Sum2/2
  Gain2/1 -> Sum2/1
  Sum2/1 -> Gain1/1
  Pe/1 -> Sum2/3
  dPm/1 -> Sum2/4

== system M10B39_es_V3/Genrators/Generator4/Output ==
  Igxy1in : Inport
  GBxyin : Inport  Port=2
  deltain : Inport  Port=3
  Pein : Inport  Port=4
  fin : Inport  Port=5
  Vg : Inport  Port=6
  Bus Creator : BusCreator  Inputs=6
  m : Outport
  Igxy1 : Outport  Port=2
  GBxy : Outport  Port=3
  wires:
  Vg/1 -> Bus Creator/6  "Vg"
  fin/1 -> Bus Creator/5  "f"
  Pein/1 -> Bus Creator/4  "Pe"
  deltain/1 -> Bus Creator/3  "delta"
  GBxyin/1 -> Bus Creator/2, GBxy/1  "GBxy"
  Igxy1in/1 -> Bus Creator/1, Igxy1/1  "Igxy1"
  Bus Creator/1 -> m/1

== system M10B39_es_V3/Genrators/Generator4/PSS1 ==
  w : Inport
  Trip : Inport  Port=2
  CT : Constant  Value=0
  Constant : Constant  Value=0
  Gain : Gain  Gain=Kpss  SaturateOnIntegerOverflow=on  OutDataTypeStr=Inherit: Same as input  ParamDataTypeStr=Inherit: Same as input
  Saturation : Saturate  UpperLimit=Upmax  LowerLimit=Upmin
  Sum3 : Sum  Inputs=|+-  SaturateOnIntegerOverflow=on
  Switch : Switch  Threshold=0.5  InputSameDT=off
  Switch1 : Switch  Threshold=0.5  InputSameDT=off
  Transfer Fcn : TransferFcn  Numerator=[Tw_P 0]  Denominator=[Tw_P 1]
  Transfer Fcn1 : TransferFcn  Numerator=[T1_P 1]  Denominator=[T2_P 1]
  Transfer Fcn2 : TransferFcn  Numerator=[T3_P 1]  Denominator=[T4_P 1]
  w0 : Constant
  w1 : Constant  Value=S_PSS
  Upss : Outport
  wires:
  Constant/1 -> Switch1/1
  Trip/1 -> Switch1/2
  Switch1/1 -> Upss/1
  Switch/1 -> Switch1/3
  Transfer Fcn/1 -> Transfer Fcn1/1
  Gain/1 -> Transfer Fcn/1
  w1/1 -> Switch/2
  CT/1 -> Switch/3
  Saturation/1 -> Switch/1
  Sum3/1 -> Gain/1
  Transfer Fcn2/1 -> Saturation/1
  Transfer Fcn1/1 -> Transfer Fcn2/1
  w/1 -> Sum3/1
  w0/1 -> Sum3/2

== system M10B39_es_V3/Genrators/Generator7/Excitation System ST1A1 ==
  note: Ef
  Upss : Inport
  Trip : Inport  Port=2
  Vg : Inport  Port=3
  Constant1 : Constant  Value=0
  Ef1 : Integrator  InitialCondition=Ef10
  K : Gain  Gain=1/Tb  SaturateOnIntegerOverflow=on  OutDataTypeStr=Inherit: Same as input  ParamDataTypeStr=Inherit: Same as input
  KA : Gain  Gain=Ka  SaturateOnIntegerOverflow=on  OutDataTypeStr=Inherit: Same as input  ParamDataTypeStr=Inherit: Same as input
  KA1 : Gain  Gain=Tc/Tb  SaturateOnIntegerOverflow=on  OutDataTypeStr=Inherit: Same as input  ParamDataTypeStr=Inherit: Same as input
  KA2 : Gain  Gain=(1/Tb)*(1-Tc/Tb)  SaturateOnIntegerOverflow=on  OutDataTypeStr=Inherit: Same as input  ParamDataTypeStr=Inherit: Same as input
  Saturation : Saturate  UpperLimit=Efmax  LowerLimit=Efmin
  Sum : Sum  Inputs=|++  SaturateOnIntegerOverflow=on
  Sum1 : Sum  Inputs=|+-  SaturateOnIntegerOverflow=on
  Sum4 : Sum  Inputs=|+-+  SaturateOnIntegerOverflow=on
  Switch2 : Switch  Criteria=u2 ~= 0  Threshold=0.5  InputSameDT=off
  Switch3 : Switch  Criteria=u2 ~= 0  Threshold=0.5  InputSameDT=off
  Vref : Constant  Value=Vref
  Ef : Outport
  wires:
  Trip/1 -> Switch3/2, Switch2/2
  Constant1/1 -> Switch3/1, Switch2/1
  Switch3/1 -> KA2/1, K/1
  Ef1/1 -> Switch3/3
  Switch2/1 -> Ef1/1
  Sum1/1 -> Switch2/3
  KA/1 -> KA1/1, Sum1/1
  Upss/1 -> Sum4/3
  Saturation/1 -> Ef/1
  Vg/1 -> Sum4/2
  Sum4/1 -> KA/1
  Vref/1 -> Sum4/1
  Sum/1 -> Saturation/1
  K/1 -> Sum1/2
  KA1/1 -> Sum/2
  KA2/1 -> Sum/1

== system M10B39_es_V3/Genrators/Generator7/Governor ==
  w : Inport
  Trip : Inport  Port=2
  CT : Constant  Value=0
  Constant : Constant  Value=0
  Gain : Gain  Gain=a_G  SaturateOnIntegerOverflow=on  OutDataTypeStr=Inherit: Same as input  ParamDataTypeStr=Inherit: Same as input
  Saturation : Saturate  UpperLimit=dPmax  LowerLimit=dPmin
  Sum1 : Sum  Inputs=|++  SaturateOnIntegerOverflow=on
  Sum3 : Sum  Inputs=|+-  SaturateOnIntegerOverflow=on
  Switch : Switch  Threshold=0.5  InputSameDT=off
  Switch1 : Switch  Criteria=u2 ~= 0  Threshold=0.5  InputSameDT=off
  Transfer Fcn1 : TransferFcn  Numerator=[b_G]  Denominator=[Tg_G 1]
  w0 : Gain  Gain=wB  SaturateOnIntegerOverflow=on  OutDataTypeStr=Inherit: Same as input  ParamDataTypeStr=Inherit: Same as input
  w1 : Constant  Value=S_Gov
  wref : Constant
  dPm : Outport
  wires:
  Gain/1 -> Sum1/1
  w1/1 -> Switch/2
  CT/1 -> Switch/3
  Sum3/1 -> w0/1
  Sum1/1 -> Saturation/1
  Saturation/1 -> Switch/1
  wref/1 -> Sum3/1
  w0/1 -> Gain/1, Transfer Fcn1/1
  Transfer Fcn1/1 -> Sum1/2
  w/1 -> Sum3/2
  Constant/1 -> Switch1/1
  Switch/1 -> Switch1/3
  Trip/1 -> Switch1/2
  Switch1/1 -> dPm/1

== system M10B39_es_V3/Genrators/Generator7/Machine Equations  ==
  note: Iqg
  note: Idg
  note: 接口
  delta : Inport
  Vgxy : Inport  Port=2
  Ef : Inport  Port=3
  Trip : Inport  Port=4
  Demux : Demux  Outputs=2
  Demux1 : Demux  Outputs=2
  Fcn1 : Fcn  Expr=u(1)*u(3)+u(2)*u(4)
  Fcn2 : Fcn  Expr=(u(3)-u(2))/Xd1
  Fcn3 : Fcn  Expr=(u(1)-u(4))/Xq1
  Fcn4 : Fcn  Expr=u(2)*u(3)-u(1)*u(4)
  Fcn6 : Fcn  Expr=sqrt(u(1)^2+u(2)^2)
  Interface : Subsystem
  Mux1 : Mux  Inputs=2
  Mux2 : Mux  Inputs=2
  Mux3 : Mux  Inputs=2
  Qe : Scope
      settings: TimeSpan=10  ActiveDisplayYMinimum=0.15  ActiveDisplayYMaximum=0.65
  Scope{,1..3} (4 alike) : Scope
      Scope settings: ActiveDisplayYMinimum=6.90941  ActiveDisplayYMaximum=6.93032
      Scope1 settings: ActiveDisplayYMinimum=0.73198  ActiveDisplayYMaximum=0.74189  DataLoggingVariableName=ScopeData2
      Scope2 settings: ActiveDisplayYMinimum=0.70724  ActiveDisplayYMaximum=0.71179  DataLoggingVariableName=ScopeData3
      Scope3 settings: ActiveDisplayYMinimum=3.59596  ActiveDisplayYMaximum=3.95434  DataLoggingVariableName=ScopeData4
  Transient Equations : Subsystem
  Pe : Outport
  Igxy1 : Outport  Port=2
  GBxy : Outport  Port=3
  Vg : Outport  Port=4
  wires:
  Trip/1 -> Transient Equations/3(Trip)
  Demux1/2 -> Scope3/1
  Demux/2 -> Scope2/1
  Demux1/1 -> Scope/1
  Demux/1 -> Scope1/1
  Transient Equations/1(Eqd') -> Interface/3(Eqd''), Mux1/2
  Interface/3(GBxy) -> GBxy/1
  Interface/2(Igxy1) -> Igxy1/1
  Vgxy/1 -> Interface/2(Vgxy)
  delta/1 -> Interface/1(delta)
  Fcn4/1 -> Qe/1
  Fcn6/1 -> Vg/1
  Fcn1/1 -> Pe/1
  Ef/1 -> Transient Equations/2(Ef)
  Mux2/1 -> Fcn4/1, Fcn1/1
  Mux1/1 -> Fcn3/1, Fcn2/1
  Interface/1(Vdqg) -> Mux1/1, Fcn6/1, Mux2/1, Demux/1
  Mux3/1 -> Mux2/2, Demux1/1, Transient Equations/1(Idqg)
  Fcn2/1 -> Mux3/1
  Fcn3/1 -> Mux3/2

== system M10B39_es_V3/Genrators/Generator7/Mechanical DE ==
  Pe : Inport
  dPm : Inport  Port=2
  Trip : Inport  Port=3
  Constant1 : Constant  Value=0
  Constant2 : Constant  Value=0
  Gain : Gain  Gain=wB  SaturateOnIntegerOverflow=on  OutDataTypeStr=Inherit: Same as input  ParamDataTypeStr=Inherit: Same as input
  Gain1 : Gain  Gain=1/H  SaturateOnIntegerOverflow=on  OutDataTypeStr=Inherit: Same as input  ParamDataTypeStr=Inherit: Same as input
  Gain2 : Gain  Gain=D  SaturateOnIntegerOverflow=on  OutDataTypeStr=Inherit: Same as input  ParamDataTypeStr=Inherit: Same as input
  Gain5 : Gain  Gain=180/pi  SaturateOnIntegerOverflow=on  OutDataTypeStr=Inherit: Same as input  ParamDataTypeStr=Inherit: Same as input
  Int1 : Integrator  InitialCondition=delta0
  Int2 : Integrator  InitialCondition=w0
  Pm : Constant  Value=Pm0
  Scope2 : Scope
      settings: TimeSpan=10  ActiveDisplayYMinimum=-0.4  ActiveDisplayYMaximum=1.4  DataLoggingVariableName=ScopeData5
  Scope4 : Scope
      settings: TimeSpan=10  ActiveDisplayYMinimum=0.99397  ActiveDisplayYMaximum=1.02044  DataLoggingVariableName=ScopeData6
  Scope8 : Scope
      settings: TimeSpan=10  ActiveDisplayYMinimum=-0.4  ActiveDisplayYMaximum=1.4  DataLoggingVariableName=ScopeData11
  Sum2 : Sum  Inputs=-+-+  SaturateOnIntegerOverflow=on
  Sum3 : Sum  Inputs=|+-  SaturateOnIntegerOverflow=on
  Switch{1..4} (4 alike) : Switch  Criteria=u2 ~= 0  Threshold=0.5  InputSameDT=off
  w0 : Constant
  delta : Outport
  w : Outport  Port=2
  wires:
  [Trip] -> Switch3/2, Switch2/2
  Constant1/1 -> Switch3/1, Switch2/1
  Switch3/1 -> Scope4/1, Sum3/1, w/1
  Int2/1 -> Switch3/3
  Switch2/1 -> Int2/1
  Gain1/1 -> Switch2/3
  Trip/1 -> [Trip]
  [Trip] -> Switch1/2, Switch4/2
  Constant2/1 -> Switch4/1, Switch1/1
  Switch4/1 -> delta/1, Scope2/1, Gain5/1
  Int1/1 -> Switch4/3
  Switch1/1 -> Int1/1
  Gain/1 -> Switch1/3
  Gain5/1 -> Scope8/1
  w0/1 -> Sum3/2
  Sum3/1 -> Gain2/1, Gain/1
  Pm/1 -> Sum2/2
  Gain2/1 -> Sum2/1
  Sum2/1 -> Gain1/1
  Pe/1 -> Sum2/3
  dPm/1 -> Sum2/4

== system M10B39_es_V3/Genrators/Generator7/Output ==
  Igxy1in : Inport
  GBxyin : Inport  Port=2
  deltain : Inport  Port=3
  Pein : Inport  Port=4
  fin : Inport  Port=5
  Vg : Inport  Port=6
  Bus Creator : BusCreator  Inputs=6
  m : Outport
  Igxy1 : Outport  Port=2
  GBxy : Outport  Port=3
  wires:
  Vg/1 -> Bus Creator/6  "Vg"
  fin/1 -> Bus Creator/5  "f"
  Pein/1 -> Bus Creator/4  "Pe"
  deltain/1 -> Bus Creator/3  "delta"
  GBxyin/1 -> Bus Creator/2, GBxy/1  "GBxy"
  Igxy1in/1 -> Bus Creator/1, Igxy1/1  "Igxy1"
  Bus Creator/1 -> m/1

== system M10B39_es_V3/Genrators/Generator7/PSS1 ==
  w : Inport
  Trip : Inport  Port=2
  CT : Constant  Value=0
  Constant : Constant  Value=0
  Gain : Gain  Gain=Kpss  SaturateOnIntegerOverflow=on  OutDataTypeStr=Inherit: Same as input  ParamDataTypeStr=Inherit: Same as input
  Saturation : Saturate  UpperLimit=Upmax  LowerLimit=Upmin
  Sum3 : Sum  Inputs=|+-  SaturateOnIntegerOverflow=on
  Switch : Switch  Threshold=0.5  InputSameDT=off
  Switch1 : Switch  Threshold=0.5  InputSameDT=off
  Transfer Fcn : TransferFcn  Numerator=[Tw_P 0]  Denominator=[Tw_P 1]
  Transfer Fcn1 : TransferFcn  Numerator=[T1_P 1]  Denominator=[T2_P 1]
  Transfer Fcn2 : TransferFcn  Numerator=[T3_P 1]  Denominator=[T4_P 1]
  w0 : Constant
  w1 : Constant  Value=S_PSS
  Upss : Outport
  wires:
  Constant/1 -> Switch1/1
  Trip/1 -> Switch1/2
  Switch1/1 -> Upss/1
  Switch/1 -> Switch1/3
  Transfer Fcn/1 -> Transfer Fcn1/1
  Gain/1 -> Transfer Fcn/1
  w1/1 -> Switch/2
  CT/1 -> Switch/3
  Saturation/1 -> Switch/1
  Sum3/1 -> Gain/1
  Transfer Fcn2/1 -> Saturation/1
  Transfer Fcn1/1 -> Transfer Fcn2/1
  w/1 -> Sum3/1
  w0/1 -> Sum3/2

== system M10B39_es_V3/Genrators/Generator9/Excitation System ST1A1 ==
  note: Ef
  Upss : Inport
  Trip : Inport  Port=2
  Vg : Inport  Port=3
  Constant1 : Constant  Value=0
  Ef1 : Integrator  InitialCondition=Ef10
  K : Gain  Gain=1/Tb  SaturateOnIntegerOverflow=on  OutDataTypeStr=Inherit: Same as input  ParamDataTypeStr=Inherit: Same as input
  KA : Gain  Gain=Ka  SaturateOnIntegerOverflow=on  OutDataTypeStr=Inherit: Same as input  ParamDataTypeStr=Inherit: Same as input
  KA1 : Gain  Gain=Tc/Tb  SaturateOnIntegerOverflow=on  OutDataTypeStr=Inherit: Same as input  ParamDataTypeStr=Inherit: Same as input
  KA2 : Gain  Gain=(1/Tb)*(1-Tc/Tb)  SaturateOnIntegerOverflow=on  OutDataTypeStr=Inherit: Same as input  ParamDataTypeStr=Inherit: Same as input
  Saturation : Saturate  UpperLimit=Efmax  LowerLimit=Efmin
  Sum : Sum  Inputs=|++  SaturateOnIntegerOverflow=on
  Sum1 : Sum  Inputs=|+-  SaturateOnIntegerOverflow=on
  Sum4 : Sum  Inputs=|+-+  SaturateOnIntegerOverflow=on
  Switch2 : Switch  Criteria=u2 ~= 0  Threshold=0.5  InputSameDT=off
  Switch3 : Switch  Criteria=u2 ~= 0  Threshold=0.5  InputSameDT=off
  Vref : Constant  Value=Vref
  Ef : Outport
  wires:
  Trip/1 -> Switch3/2, Switch2/2
  Constant1/1 -> Switch3/1, Switch2/1
  Switch3/1 -> KA2/1, K/1
  Ef1/1 -> Switch3/3
  Switch2/1 -> Ef1/1
  Sum1/1 -> Switch2/3
  KA/1 -> KA1/1, Sum1/1
  Upss/1 -> Sum4/3
  Saturation/1 -> Ef/1
  Vg/1 -> Sum4/2
  Sum4/1 -> KA/1
  Vref/1 -> Sum4/1
  Sum/1 -> Saturation/1
  K/1 -> Sum1/2
  KA1/1 -> Sum/2
  KA2/1 -> Sum/1

== system M10B39_es_V3/Genrators/Generator9/Governor ==
  w : Inport
  Trip : Inport  Port=2
  CT : Constant  Value=0
  Constant : Constant  Value=0
  Gain : Gain  Gain=a_G  SaturateOnIntegerOverflow=on  OutDataTypeStr=Inherit: Same as input  ParamDataTypeStr=Inherit: Same as input
  Saturation : Saturate  UpperLimit=dPmax  LowerLimit=dPmin
  Sum1 : Sum  Inputs=|++  SaturateOnIntegerOverflow=on
  Sum3 : Sum  Inputs=|+-  SaturateOnIntegerOverflow=on
  Switch : Switch  Threshold=0.5  InputSameDT=off
  Switch1 : Switch  Criteria=u2 ~= 0  Threshold=0.5  InputSameDT=off
  Transfer Fcn1 : TransferFcn  Numerator=[b_G]  Denominator=[Tg_G 1]
  w0 : Gain  Gain=wB  SaturateOnIntegerOverflow=on  OutDataTypeStr=Inherit: Same as input  ParamDataTypeStr=Inherit: Same as input
  w1 : Constant  Value=S_Gov
  wref : Constant
  dPm : Outport
  wires:
  Gain/1 -> Sum1/1
  w1/1 -> Switch/2
  CT/1 -> Switch/3
  Sum3/1 -> w0/1
  Sum1/1 -> Saturation/1
  Saturation/1 -> Switch/1
  wref/1 -> Sum3/1
  w0/1 -> Gain/1, Transfer Fcn1/1
  Transfer Fcn1/1 -> Sum1/2
  w/1 -> Sum3/2
  Constant/1 -> Switch1/1
  Switch/1 -> Switch1/3
  Trip/1 -> Switch1/2
  Switch1/1 -> dPm/1

== system M10B39_es_V3/Genrators/Generator9/Machine Equations  ==
  note: Iqg
  note: Idg
  note: 接口
  delta : Inport
  Vgxy : Inport  Port=2
  Ef : Inport  Port=3
  Trip : Inport  Port=4
  Demux : Demux  Outputs=2
  Demux1 : Demux  Outputs=2
  Fcn1 : Fcn  Expr=u(1)*u(3)+u(2)*u(4)
  Fcn2 : Fcn  Expr=(u(3)-u(2))/Xd1
  Fcn3 : Fcn  Expr=(u(1)-u(4))/Xq1
  Fcn4 : Fcn  Expr=u(2)*u(3)-u(1)*u(4)
  Fcn6 : Fcn  Expr=sqrt(u(1)^2+u(2)^2)
  Interface : Subsystem
  Mux1 : Mux  Inputs=2
  Mux2 : Mux  Inputs=2
  Mux3 : Mux  Inputs=2
  Qe : Scope
      settings: TimeSpan=10  ActiveDisplayYMinimum=0.15  ActiveDisplayYMaximum=0.65
  Scope{,1..3} (4 alike) : Scope
      Scope settings: ActiveDisplayYMinimum=6.90941  ActiveDisplayYMaximum=6.93032
      Scope1 settings: ActiveDisplayYMinimum=0.73198  ActiveDisplayYMaximum=0.74189  DataLoggingVariableName=ScopeData2
      Scope2 settings: ActiveDisplayYMinimum=0.70724  ActiveDisplayYMaximum=0.71179  DataLoggingVariableName=ScopeData3
      Scope3 settings: ActiveDisplayYMinimum=3.59596  ActiveDisplayYMaximum=3.95434  DataLoggingVariableName=ScopeData4
  Transient Equations : Subsystem
  Pe : Outport
  Igxy1 : Outport  Port=2
  GBxy : Outport  Port=3
  Vg : Outport  Port=4
  wires:
  Trip/1 -> Transient Equations/3(Trip)
  Demux1/2 -> Scope3/1
  Demux/2 -> Scope2/1
  Demux1/1 -> Scope/1
  Demux/1 -> Scope1/1
  Transient Equations/1(Eqd') -> Interface/3(Eqd''), Mux1/2
  Interface/3(GBxy) -> GBxy/1
  Interface/2(Igxy1) -> Igxy1/1
  Vgxy/1 -> Interface/2(Vgxy)
  delta/1 -> Interface/1(delta)
  Fcn4/1 -> Qe/1
  Fcn6/1 -> Vg/1
  Fcn1/1 -> Pe/1
  Ef/1 -> Transient Equations/2(Ef)
  Mux2/1 -> Fcn4/1, Fcn1/1
  Mux1/1 -> Fcn3/1, Fcn2/1
  Interface/1(Vdqg) -> Mux1/1, Fcn6/1, Mux2/1, Demux/1
  Mux3/1 -> Mux2/2, Demux1/1, Transient Equations/1(Idqg)
  Fcn2/1 -> Mux3/1
  Fcn3/1 -> Mux3/2

== system M10B39_es_V3/Genrators/Generator9/Mechanical DE ==
  Pe : Inport
  dPm : Inport  Port=2
  Trip : Inport  Port=3
  Constant1 : Constant  Value=0
  Constant2 : Constant  Value=0
  Gain : Gain  Gain=wB  SaturateOnIntegerOverflow=on  OutDataTypeStr=Inherit: Same as input  ParamDataTypeStr=Inherit: Same as input
  Gain1 : Gain  Gain=1/H  SaturateOnIntegerOverflow=on  OutDataTypeStr=Inherit: Same as input  ParamDataTypeStr=Inherit: Same as input
  Gain2 : Gain  Gain=D  SaturateOnIntegerOverflow=on  OutDataTypeStr=Inherit: Same as input  ParamDataTypeStr=Inherit: Same as input
  Gain5 : Gain  Gain=180/pi  SaturateOnIntegerOverflow=on  OutDataTypeStr=Inherit: Same as input  ParamDataTypeStr=Inherit: Same as input
  Int1 : Integrator  InitialCondition=delta0
  Int2 : Integrator  InitialCondition=w0
  Pm : Constant  Value=Pm0
  Scope2 : Scope
      settings: TimeSpan=10  ActiveDisplayYMinimum=-0.4  ActiveDisplayYMaximum=1.4  DataLoggingVariableName=ScopeData5
  Scope4 : Scope
      settings: TimeSpan=10  ActiveDisplayYMinimum=0.99397  ActiveDisplayYMaximum=1.02044  DataLoggingVariableName=ScopeData6
  Scope8 : Scope
      settings: TimeSpan=10  ActiveDisplayYMinimum=-0.4  ActiveDisplayYMaximum=1.4  DataLoggingVariableName=ScopeData11
  Sum2 : Sum  Inputs=-+-+  SaturateOnIntegerOverflow=on
  Sum3 : Sum  Inputs=|+-  SaturateOnIntegerOverflow=on
  Switch{1..4} (4 alike) : Switch  Criteria=u2 ~= 0  Threshold=0.5  InputSameDT=off
  w0 : Constant
  delta : Outport
  w : Outport  Port=2
  wires:
  [Trip] -> Switch3/2, Switch2/2
  Constant1/1 -> Switch3/1, Switch2/1
  Switch3/1 -> Scope4/1, Sum3/1, w/1
  Int2/1 -> Switch3/3
  Switch2/1 -> Int2/1
  Gain1/1 -> Switch2/3
  Trip/1 -> [Trip]
  [Trip] -> Switch1/2, Switch4/2
  Constant2/1 -> Switch4/1, Switch1/1
  Switch4/1 -> delta/1, Scope2/1, Gain5/1
  Int1/1 -> Switch4/3
  Switch1/1 -> Int1/1
  Gain/1 -> Switch1/3
  Gain5/1 -> Scope8/1
  w0/1 -> Sum3/2
  Sum3/1 -> Gain2/1, Gain/1
  Pm/1 -> Sum2/2
  Gain2/1 -> Sum2/1
  Sum2/1 -> Gain1/1
  Pe/1 -> Sum2/3
  dPm/1 -> Sum2/4

== system M10B39_es_V3/Genrators/Generator9/Output ==
  Igxy1in : Inport
  GBxyin : Inport  Port=2
  deltain : Inport  Port=3
  Pein : Inport  Port=4
  fin : Inport  Port=5
  Vg : Inport  Port=6
  Bus Creator : BusCreator  Inputs=6
  m : Outport
  Igxy1 : Outport  Port=2
  GBxy : Outport  Port=3
  wires:
  Vg/1 -> Bus Creator/6  "Vg"
  fin/1 -> Bus Creator/5  "f"
  Pein/1 -> Bus Creator/4  "Pe"
  deltain/1 -> Bus Creator/3  "delta"
  GBxyin/1 -> Bus Creator/2, GBxy/1  "GBxy"
  Igxy1in/1 -> Bus Creator/1, Igxy1/1  "Igxy1"
  Bus Creator/1 -> m/1

== system M10B39_es_V3/Genrators/Generator9/PSS1 ==
  w : Inport
  Trip : Inport  Port=2
  CT : Constant  Value=0
  Constant : Constant  Value=0
  Gain : Gain  Gain=Kpss  SaturateOnIntegerOverflow=on  OutDataTypeStr=Inherit: Same as input  ParamDataTypeStr=Inherit: Same as input
  Saturation : Saturate  UpperLimit=Upmax  LowerLimit=Upmin
  Sum3 : Sum  Inputs=|+-  SaturateOnIntegerOverflow=on
  Switch : Switch  Threshold=0.5  InputSameDT=off
  Switch1 : Switch  Threshold=0.5  InputSameDT=off
  Transfer Fcn : TransferFcn  Numerator=[Tw_P 0]  Denominator=[Tw_P 1]
  Transfer Fcn1 : TransferFcn  Numerator=[T1_P 1]  Denominator=[T2_P 1]
  Transfer Fcn2 : TransferFcn  Numerator=[T3_P 1]  Denominator=[T4_P 1]
  w0 : Constant
  w1 : Constant  Value=S_PSS
  Upss : Outport
  wires:
  Constant/1 -> Switch1/1
  Trip/1 -> Switch1/2
  Switch1/1 -> Upss/1
  Switch/1 -> Switch1/3
  Transfer Fcn/1 -> Transfer Fcn1/1
  Gain/1 -> Transfer Fcn/1
  w1/1 -> Switch/2
  CT/1 -> Switch/3
  Saturation/1 -> Switch/1
  Sum3/1 -> Gain/1
  Transfer Fcn2/1 -> Saturation/1
  Transfer Fcn1/1 -> Transfer Fcn2/1
  w/1 -> Sum3/1
  w0/1 -> Sum3/2
